simulink model "mass_spring_damper"  (R2025b)
settings: Solver=FixedStepAuto  StartTime=0.0  StopTime=10  FixedStep=0.01  RelTol=1e-3
values from neighbouring files (symbols this model uses):
  c = Simulink.Parameter(100)    [mass_spring_damper_script.m]
  d = Simulink.Parameter(5)    [mass_spring_damper_script.m]
  m = Simulink.Parameter(1)    [mass_spring_damper_script.m]
settings Model: Creator=fycce  LastModifiedBy=fycce

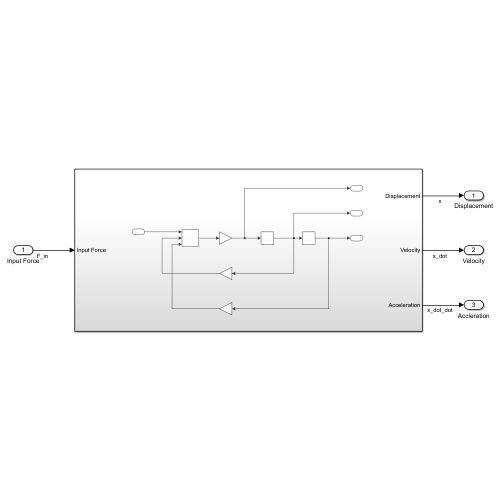
[thumbnail: Simulink's stored preview of the top-level diagram]
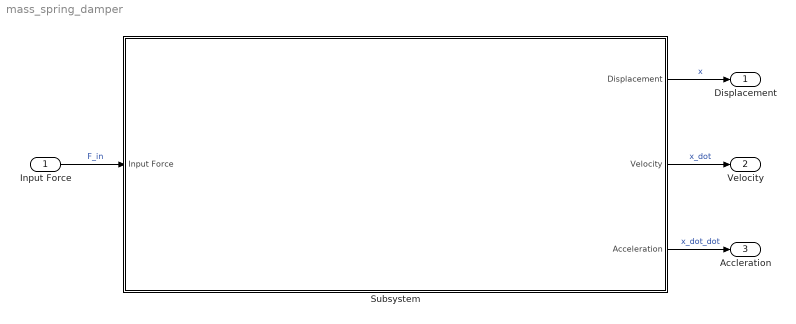
== system mass_spring_damper ==
  Input Force : Inport
  Subsystem : Subsystem
  Displacement : Outport
  Velocity : Outport  Port=2
  Accleration : Outport  Port=3
  wires:
  Input Force/1 -> Subsystem/1(Input Force)  "F_in"
  Subsystem/1(Displacement) -> Displacement/1  "x"
  Subsystem/2(Velocity) -> Velocity/1  "x_dot"
  Subsystem/3(Acceleration) -> Accleration/1  "x_dot_dot"

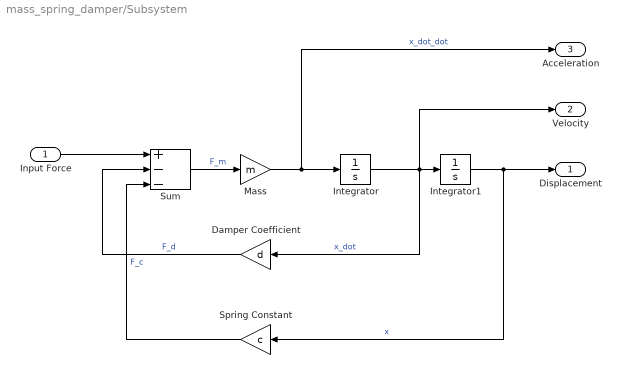
== system mass_spring_damper/Subsystem ==
  Input Force : Inport
  Damper Coefficient : Gain  Gain=d
  Integrator : Integrator
  Integrator1 : Integrator
  Mass : Gain  Gain=m
  Spring Constant : Gain  Gain=c
  Sum : Sum  Inputs=+--
  Displacement : Outport
  Velocity : Outport  Port=2
  Acceleration : Outport  Port=3
  wires:
  Integrator/1 -> Velocity/1, Integrator1/1, Damper Coefficient/1  "x_dot"
  Integrator1/1 -> Displacement/1, Spring Constant/1  "x"
  Spring Constant/1 -> Sum/3  "F_c"
  Input Force/1 -> Sum/1
  Mass/1 -> Integrator/1, Acceleration/1  "x_dot_dot"
  Damper Coefficient/1 -> Sum/2  "F_d"
  Sum/1 -> Mass/1  "F_m"
